simulink model "TEP_Final_NoScript"  (R2024a)
settings: Solver=FixedStepAuto  StartTime=0.0  StopTime=10  FixedStep=1/3600  RelTol=1e-3
model workspace (MAT data in the model file):
  AD : Simulink.Parameter (value not decoded)
  AG : Simulink.Parameter (value not decoded)
  AH : Simulink.Parameter (value not decoded)
  AV : Simulink.Parameter (value not decoded)
  AVP : Simulink.Parameter (value not decoded)
  BCHL : Simulink.Parameter (value not decoded)
  BCHV : Simulink.Parameter (value not decoded)
  BD : Simulink.Parameter (value not decoded)
  BG : Simulink.Parameter (value not decoded)
  BH : Simulink.Parameter (value not decoded)
  BVP : Simulink.Parameter (value not decoded)
  CD : Simulink.Parameter (value not decoded)
  CG : Simulink.Parameter (value not decoded)
  CH : Simulink.Parameter (value not decoded)
  CVP : Simulink.Parameter (value not decoded)
  XMW : Simulink.Parameter (value not decoded)
  XNS : Simulink.Parameter (value not decoded)
  XNSE : Simulink.Parameter (value not decoded)
symbols that are objects in the model workspace (value not decoded): AD, AG, AH, AV, AVP, BD, BG, BH, BVP, CD, CG, CH, CVP, XMW, XNS, XNSE
undefined symbols (not defined in the file or in its folder): magnitude, msgbox, SETPT, XMEAS, XMV
libraries: mylib x360, dspindex x28
(part 7 of 14)

== system TEP_Final_NoScript/Separator/Holdup of Components in Separator/Subsystem3 ==
  Bus Creator : BusCreator  Inputs=8
  Bus Selector3 : BusSelector  OutputSignals=signal1.FCM(I;11)
  FCM(1,11) : Gain
  FCM(2,11) : Gain
  FCM(3,11) : Gain
  FCM(4,11) : Gain
  FCM(5,11) : Gain
  FCM(6,11) : Gain
  FCM(7,11) : Gain
  FCM(8,11) : Gain
  Multiport Selector3 : dspindex/Multiport Selector  rowsOrCols=Rows  idxCellArray={1,2,3,4,5,6,7,8}  idxErrMode=Clip Index
  FCM(I;11) : Outport  VectorParamsAs1DForOutWhenUnconnected=off
  wires:
  Multiport Selector3/3 -> FCM(3,11)/1
  Multiport Selector3/2 -> FCM(2,11)/1
  Multiport Selector3/5 -> FCM(5,11)/1
  Multiport Selector3/8 -> FCM(8,11)/1
  Bus Selector3/1 -> Multiport Selector3/1  "<FCM(I;11)>"
  Multiport Selector3/7 -> FCM(7,11)/1
  Multiport Selector3/6 -> FCM(6,11)/1
  Multiport Selector3/1 -> FCM(1,11)/1
  Multiport Selector3/4 -> FCM(4,11)/1
  [PropertiesStream11] -> Bus Selector3/1
  FCM(5,11)/1 -> Bus Creator/5  "FCM(5;11)"
  FCM(8,11)/1 -> Bus Creator/8  "FCM(8;11)"
  FCM(7,11)/1 -> Bus Creator/7  "FCM(7;11)"
  FCM(6,11)/1 -> Bus Creator/6  "FCM(6;11)"
  FCM(2,11)/1 -> Bus Creator/2  "FCM(2;11)"
  FCM(3,11)/1 -> Bus Creator/3  "FCM(3;11)"
  FCM(4,11)/1 -> Bus Creator/4  "FCM(4;11)"
  FCM(1,11)/1 -> Bus Creator/1  "FCM(1;11)"
  Bus Creator/1 -> FCM(I;11)/1

== system TEP_Final_NoScript/Separator/Holdup of Components in Separator/YP(10) ==
  FCM(1,8) : Inport
  FCM(1,9) : Inport  Port=2
  FCM(1,10) : Inport  Port=3
  FCM(1,11) : Inport  Port=4
  " " : Sum  Inputs=+---
  Bus Selector : BusSelector  OutputSignals=FCM(1;8)
  Bus Selector1 : BusSelector  OutputSignals=FCM(1;9)
  Bus Selector2 : BusSelector  OutputSignals=FCM(1;10)
  Bus Selector3 : BusSelector  OutputSignals=FCM(1;11)
  Integration : mylib/Integration  SystemSampleTime=-1  VariantActivationTime=update diagram  AllowFlexibleInterface=on  Latency=0  AutoFrameSizeCalculation=off
      settings: SourceProductName=TEP Library
  "YY(10) " : Constant  Value=63.75581199
  YY(10) : Outport  VectorParamsAs1DForOutWhenUnconnected=off
  wires:
  "YY(10) "/1 -> Integration/2
  FCM(1,10)/1 -> Bus Selector2/1
  FCM(1,9)/1 -> Bus Selector1/1
  FCM(1,8)/1 -> Bus Selector/1
  " "/1 -> Integration/1
  Integration/1 -> YY(10)/1
  FCM(1,11)/1 -> Bus Selector3/1
  Bus Selector/1 -> " "/1  "<FCM(1;8)>"
  Bus Selector1/1 -> " "/2  "<FCM(1;9)>"
  Bus Selector2/1 -> " "/3  "<FCM(1;10)>"
  Bus Selector3/1 -> " "/4  "<FCM(1;11)>"

== system TEP_Final_NoScript/Separator/Holdup of Components in Separator/YP(11) ==
  FCM(2,8) : Inport
  FCM(2,9) : Inport  Port=2
  FCM(2,10) : Inport  Port=3
  FCM(2,11) : Inport  Port=4
  " " : Sum  Inputs=+---
  Bus Selector : BusSelector  OutputSignals=FCM(2;8)
  Bus Selector1 : BusSelector  OutputSignals=FCM(2;9)
  Bus Selector2 : BusSelector  OutputSignals=FCM(2;10)
  Bus Selector3 : BusSelector  OutputSignals=FCM(2;11)
  Integration : mylib/Integration  SystemSampleTime=-1  VariantActivationTime=update diagram  AllowFlexibleInterface=on  Latency=0  AutoFrameSizeCalculation=off
      settings: SourceProductName=TEP Library
  "YY(11) " : Constant  Value=26.74026066
  YY(11) : Outport  VectorParamsAs1DForOutWhenUnconnected=off
  wires:
  Integration/1 -> YY(11)/1
  FCM(2,8)/1 -> Bus Selector/1
  FCM(2,9)/1 -> Bus Selector1/1
  FCM(2,10)/1 -> Bus Selector2/1
  FCM(2,11)/1 -> Bus Selector3/1
  "YY(11) "/1 -> Integration/2
  " "/1 -> Integration/1
  Bus Selector/1 -> " "/1  "<FCM(2;8)>"
  Bus Selector1/1 -> " "/2  "<FCM(2;9)>"
  Bus Selector2/1 -> " "/3  "<FCM(2;10)>"
  Bus Selector3/1 -> " "/4  "<FCM(2;11)>"

== system TEP_Final_NoScript/Separator/Holdup of Components in Separator/YP(12) ==
  FCM(3,8) : Inport
  FCM(3,9) : Inport  Port=2
  FCM(3,10) : Inport  Port=3
  FCM(3,11) : Inport  Port=4
  " " : Sum  Inputs=+---
  Bus Selector : BusSelector  OutputSignals=FCM(3;11)
  Bus Selector1 : BusSelector  OutputSignals=FCM(3;10)
  Bus Selector2 : BusSelector  OutputSignals=FCM(3;9)
  Bus Selector3 : BusSelector  OutputSignals=FCM(3;8)
  Integration : mylib/Integration  SystemSampleTime=-1  VariantActivationTime=update diagram  AllowFlexibleInterface=on  Latency=0  AutoFrameSizeCalculation=off
      settings: SourceProductName=TEP Library
  "YY(12) " : Constant  Value=46.38532432
  YY(12) : Outport  VectorParamsAs1DForOutWhenUnconnected=off
  wires:
  Integration/1 -> YY(12)/1
  FCM(3,8)/1 -> Bus Selector3/1
  FCM(3,9)/1 -> Bus Selector2/1
  FCM(3,10)/1 -> Bus Selector1/1
  FCM(3,11)/1 -> Bus Selector/1
  " "/1 -> Integration/1
  "YY(12) "/1 -> Integration/2
  Bus Selector3/1 -> " "/1  "<FCM(3;8)>"
  Bus Selector2/1 -> " "/2  "<FCM(3;9)>"
  Bus Selector1/1 -> " "/3  "<FCM(3;10)>"
  Bus Selector/1 -> " "/4  "<FCM(3;11)>"

== system TEP_Final_NoScript/Separator/Holdup of Components in Separator/YP(13) ==
  FCM(4,8) : Inport
  FCM(4,9) : Inport  Port=2
  FCM(4,10) : Inport  Port=3
  FCM(4,11) : Inport  Port=4
  " " : Sum  Inputs=+---
  Bus Selector : BusSelector  OutputSignals=FCM(4;11)
  Bus Selector1 : BusSelector  OutputSignals=FCM(4;10)
  Bus Selector2 : BusSelector  OutputSignals=FCM(4;9)
  Bus Selector3 : BusSelector  OutputSignals=FCM(4;8)
  Integration : mylib/Integration  SystemSampleTime=-1  VariantActivationTime=update diagram  AllowFlexibleInterface=on  Latency=0  AutoFrameSizeCalculation=off
      settings: SourceProductName=TEP Library
  YY(13) : Constant  Value=0.2464521543
  "YY(13) " : Outport  VectorParamsAs1DForOutWhenUnconnected=off
  wires:
  Integration/1 -> "YY(13) "/1
  FCM(4,8)/1 -> Bus Selector3/1
  FCM(4,9)/1 -> Bus Selector2/1
  FCM(4,10)/1 -> Bus Selector1/1
  FCM(4,11)/1 -> Bus Selector/1
  " "/1 -> Integration/1
  YY(13)/1 -> Integration/2
  Bus Selector3/1 -> " "/1  "<FCM(4;8)>"
  Bus Selector2/1 -> " "/2  "<FCM(4;9)>"
  Bus Selector1/1 -> " "/3  "<FCM(4;10)>"
  Bus Selector/1 -> " "/4  "<FCM(4;11)>"

== system TEP_Final_NoScript/Separator/Holdup of Components in Separator/YP(14) ==
  FCM(5,8) : Inport
  FCM(5,9) : Inport  Port=2
  FCM(5,10) : Inport  Port=3
  FCM(5,11) : Inport  Port=4
  " " : Sum  Inputs=+---
  Bus Selector : BusSelector  OutputSignals=FCM(5;8)
  Bus Selector1 : BusSelector  OutputSignals=FCM(5;9)
  Bus Selector2 : BusSelector  OutputSignals=FCM(5;11)
  Bus Selector3 : BusSelector  OutputSignals=FCM(5;10)
  Integration : mylib/Integration  SystemSampleTime=-1  VariantActivationTime=update diagram  AllowFlexibleInterface=on  Latency=0  AutoFrameSizeCalculation=off
      settings: SourceProductName=TEP Library
  YY(14) : Constant  Value=15.20484404
  "YY(14) " : Outport  VectorParamsAs1DForOutWhenUnconnected=off
  wires:
  Integration/1 -> "YY(14) "/1
  FCM(5,8)/1 -> Bus Selector/1
  FCM(5,9)/1 -> Bus Selector1/1
  FCM(5,10)/1 -> Bus Selector3/1
  FCM(5,11)/1 -> Bus Selector2/1
  " "/1 -> Integration/1
  YY(14)/1 -> Integration/2
  Bus Selector/1 -> " "/1  "<FCM(5;8)>"
  Bus Selector1/1 -> " "/2  "<FCM(5;9)>"
  Bus Selector3/1 -> " "/3  "<FCM(5;10)>"
  Bus Selector2/1 -> " "/4  "<FCM(5;11)>"

== system TEP_Final_NoScript/Separator/Holdup of Components in Separator/YP(15) ==
  FCM(6,8) : Inport
  FCM(6,9) : Inport  Port=2
  FCM(6,10) : Inport  Port=3
  FCM(6,11) : Inport  Port=4
  " " : Sum  Inputs=+---
  Bus Selector : BusSelector  OutputSignals=FCM(6;8)
  Bus Selector1 : BusSelector  OutputSignals=FCM(6;11)
  Bus Selector2 : BusSelector  OutputSignals=FCM(6;10)
  Bus Selector3 : BusSelector  OutputSignals=FCM(6;9)
  Integration : mylib/Integration  SystemSampleTime=-1  VariantActivationTime=update diagram  AllowFlexibleInterface=on  Latency=0  AutoFrameSizeCalculation=off
      settings: SourceProductName=TEP Library
  YY(15) : Constant  Value=1.852266172
  "YY(15) " : Outport  VectorParamsAs1DForOutWhenUnconnected=off
  wires:
  Integration/1 -> "YY(15) "/1
  FCM(6,8)/1 -> Bus Selector/1
  FCM(6,9)/1 -> Bus Selector3/1
  FCM(6,10)/1 -> Bus Selector2/1
  FCM(6,11)/1 -> Bus Selector1/1
  " "/1 -> Integration/1
  YY(15)/1 -> Integration/2
  Bus Selector3/1 -> " "/2  "<FCM(6;9)>"
  Bus Selector2/1 -> " "/3  "<FCM(6;10)>"
  Bus Selector1/1 -> " "/4  "<FCM(6;11)>"
  Bus Selector/1 -> " "/1  "<FCM(6;8)>"

== system TEP_Final_NoScript/Separator/Holdup of Components in Separator/YP(16) ==
  FCM(7,8) : Inport
  FCM(7,9) : Inport  Port=2
  FCM(7,10) : Inport  Port=3
  FCM(7,11) : Inport  Port=4
  " " : Sum  Inputs=+---
  Bus Selector : BusSelector  OutputSignals=FCM(7;11)
  Bus Selector1 : BusSelector  OutputSignals=FCM(7;10)
  Bus Selector2 : BusSelector  OutputSignals=FCM(7;9)
  Bus Selector3 : BusSelector  OutputSignals=FCM(7;8)
  Integration : mylib/Integration  SystemSampleTime=-1  VariantActivationTime=update diagram  AllowFlexibleInterface=on  Latency=0  AutoFrameSizeCalculation=off
      settings: SourceProductName=TEP Library
  YY(16) : Constant  Value=52.44639459
  "YY(16) " : Outport  VectorParamsAs1DForOutWhenUnconnected=off
  wires:
  Integration/1 -> "YY(16) "/1
  FCM(7,8)/1 -> Bus Selector3/1
  FCM(7,9)/1 -> Bus Selector2/1
  FCM(7,10)/1 -> Bus Selector1/1
  FCM(7,11)/1 -> Bus Selector/1
  " "/1 -> Integration/1
  YY(16)/1 -> Integration/2
  Bus Selector3/1 -> " "/1  "<FCM(7;8)>"
  Bus Selector2/1 -> " "/2  "<FCM(7;9)>"
  Bus Selector1/1 -> " "/3  "<FCM(7;10)>"
  Bus Selector/1 -> " "/4  "<FCM(7;11)>"

== system TEP_Final_NoScript/Separator/Holdup of Components in Separator/YP(17) ==
  FCM(8,8) : Inport
  FCM(8,9) : Inport  Port=2
  FCM(8,10) : Inport  Port=3
  FCM(8,11) : Inport  Port=4
  " " : Sum  Inputs=+---
  Bus Selector : BusSelector  OutputSignals=FCM(8;11)
  Bus Selector1 : BusSelector  OutputSignals=FCM(8;10)
  Bus Selector2 : BusSelector  OutputSignals=FCM(8;9)
  Bus Selector3 : BusSelector  OutputSignals=FCM(8;8)
  Integration : mylib/Integration  SystemSampleTime=-1  VariantActivationTime=update diagram  AllowFlexibleInterface=on  Latency=0  AutoFrameSizeCalculation=off
      settings: SourceProductName=TEP Library
  YY(17) : Constant  Value=41.20394008
  "YY(17) " : Outport  VectorParamsAs1DForOutWhenUnconnected=off
  wires:
  Integration/1 -> "YY(17) "/1
  FCM(8,8)/1 -> Bus Selector3/1
  FCM(8,9)/1 -> Bus Selector2/1
  FCM(8,10)/1 -> Bus Selector1/1
  " "/1 -> Integration/1
  YY(17)/1 -> Integration/2
  FCM(8,11)/1 -> Bus Selector/1
  Bus Selector3/1 -> " "/1  "<FCM(8;8)>"
  Bus Selector2/1 -> " "/2  "<FCM(8;9)>"
  Bus Selector1/1 -> " "/3  "<FCM(8;10)>"
  Bus Selector/1 -> " "/4  "<FCM(8;11)>"

== system TEP_Final_NoScript/Separator/Pressure of Separator/Subsystem ==
  TCS : Inport
  VVS : Inport  Port=2
  UCVS : Inport  Port=3
  Bus Selector : BusSelector  OutputSignals=UCVS(1),UCVS(2),UCVS(3)
  PPS(1) Partial pressure of Component A mmHg : Product  Inputs=***/
  PPS(2) Partial pressure of Component B mmHg : Product  Inputs=***/
  PPS(3) Partial pressure of Component C mmHg : Product  Inputs=***/
  RG Universal Gas Constant ft³·mmHg/K·lb-mol : Constant  Value=998.9
  TKS Temperature in Separator K : Sum
  To Convert °C to K : Constant  Value=273.15
  PPS(1) : Outport  VectorParamsAs1DForOutWhenUnconnected=off
  PPS(2) : Outport  Port=2  VectorParamsAs1DForOutWhenUnconnected=off
  PPS(3) : Outport  Port=3  VectorParamsAs1DForOutWhenUnconnected=off
  wires:
  Bus Selector/3 -> PPS(3) Partial pressure of Component C mmHg/1  "<UCVS(3)>"
  RG Universal Gas Constant ft³·mmHg/K·lb-mol/1 -> PPS(3) Partial pressure of Component C mmHg/2, PPS(1) Partial pressure of Component A mmHg/2, PPS(2) Partial pressure of Component B mmHg/2
  UCVS/1 -> Bus Selector/1
  Bus Selector/1 -> PPS(1) Partial pressure of Component A mmHg/1  "<UCVS(1)>"
  Bus Selector/2 -> PPS(2) Partial pressure of Component B mmHg/1  "<UCVS(2)>"
  VVS/1 -> PPS(3) Partial pressure of Component C mmHg/4, PPS(2) Partial pressure of Component B mmHg/4, PPS(1) Partial pressure of Component A mmHg/4
  PPS(3) Partial pressure of Component C mmHg/1 -> PPS(3)/1
  To Convert °C to K/1 -> TKS Temperature in Separator K/2
  PPS(1) Partial pressure of Component A mmHg/1 -> PPS(1)/1
  TKS Temperature in Separator K/1 -> PPS(3) Partial pressure of Component C mmHg/3, PPS(2) Partial pressure of Component B mmHg/3, PPS(1) Partial pressure of Component A mmHg/3
  PPS(2) Partial pressure of Component B mmHg/1 -> PPS(2)/1
  TCS/1 -> TKS Temperature in Separator K/1

== system TEP_Final_NoScript/Separator/Pressure of Separator/VPR Vapour Pressure mmHg ==
  TCS : Inport
  AVP(I) Antoine Coefficient A ln(mmHg) : Constant  Value=AVP
  Add : Sum
  Add1 : Sum
  BVP(I) Antoine Coefficient B ln(mmHg)·°C : Constant  Value=BVP
  CVP(I) Antoine Coefficient C °C : Constant  Value=CVP
  Divide : Product  Inputs=*/
  Math Function : Math  SignedPower=on
  VPR : Outport  VectorParamsAs1DForOutWhenUnconnected=off
  wires:
  BVP(I) Antoine Coefficient B ln(mmHg)·°C/1 -> Divide/1
  CVP(I) Antoine Coefficient C °C/1 -> Add/1
  AVP(I) Antoine Coefficient A ln(mmHg)/1 -> Add1/1
  Add/1 -> Divide/2
  Divide/1 -> Add1/2
  Add1/1 -> Math Function/1
  Math Function/1 -> VPR/1
  TCS/1 -> Add/2

== system TEP_Final_NoScript/Separator/Stream 10/HST(10) Molar Enthalpy of Stream 10 MBtu//lb-mol ==
  ITY : Inport
  T : Inport  Port=2
  XST(I,I) : Inport  Port=3
  "Enthalpy of Stream " : mylib/Enthalpy of Stream   SystemSampleTime=-1  VariantActivationTime=update diagram  AllowFlexibleInterface=on  Latency=0  AutoFrameSizeCalculation=off
      settings: SourceProductName=TEP Library
  "H " : Outport  VectorParamsAs1DForOutWhenUnconnected=off
  wires:
  ITY/1 -> "Enthalpy of Stream "/1
  T/1 -> "Enthalpy of Stream "/2
  XST(I,I)/1 -> "Enthalpy of Stream "/3
  "Enthalpy of Stream "/1 -> "H "/1

== system TEP_Final_NoScript/Separator/Stream 10/Subsystem ==
  VPOS(6) : Inport  PortDimensions=1
  Abs : Abs  SaturateOnIntegerOverflow=off
  Constant : Constant  Value=0.0
  Constant1 : Constant  Value=0.151169
  Constant2 : Constant  Value=760
  DLP : Sum  Inputs=+-
  DLP Pressure drop between separator and environment : Merge
  FLMS : Product  Inputs=3
  If : If  IfExpression=u1 < 0
  If Action Subsystem : Subsystem  TreatAsAtomicUnit=on
  If Action Subsystem1 : Subsystem  TreatAsAtomicUnit=on
  Sqrt : Sqrt
  Out1 : Outport  VectorParamsAs1DForOutWhenUnconnected=off
  wires:
  Constant2/1 -> DLP/2
  Constant1/1 -> FLMS/2
  Abs/1 -> Sqrt/1
  DLP Pressure drop between separator and environment/1 -> Abs/1
  [PTS] -> DLP/1
  If Action Subsystem/1(Out1) -> DLP Pressure drop between separator and environment/1
  Constant/1 -> If Action Subsystem/1(In1)
  Sqrt/1 -> FLMS/3
  If Action Subsystem1/1(Out1) -> DLP Pressure drop between separator and environment/2
  If/2 -> If Action Subsystem1/Action
  DLP/1 -> If Action Subsystem1/1(In1), If/1
  VPOS(6)/1 -> FLMS/1
  If/1 -> If Action Subsystem/Action
  FLMS/1 -> Out1/1

== system TEP_Final_NoScript/Separator/Stream 10/XMWS(10) Molecular weight of Stream 10 lb//lb-mol ==
  XST(I,10) : Inport
  Constant : Constant  Value=XMW
  Product : Product
  Sum of Elements : Sum  Inputs=+
  XMWS(10) : Outport  VectorParamsAs1DForOutWhenUnconnected=off
  wires:
  Sum of Elements/1 -> XMWS(10)/1
  Product/1 -> Sum of Elements/1
  XST(I,10)/1 -> Product/1
  Constant/1 -> Product/2

== system TEP_Final_NoScript/Separator/Stream 11/HST(10) Molar Enthalpy of Stream 10 MBtu//lb-mol ==
  ITY : Inport
  T : Inport  Port=2
  XST(I,I) : Inport  Port=3
  "Enthalpy of Stream " : mylib/Enthalpy of Stream   SystemSampleTime=-1  VariantActivationTime=update diagram  AllowFlexibleInterface=on  Latency=0  AutoFrameSizeCalculation=off
      settings: SourceProductName=TEP Library
  "H " : Outport  VectorParamsAs1DForOutWhenUnconnected=off
  wires:
  ITY/1 -> "Enthalpy of Stream "/1
  T/1 -> "Enthalpy of Stream "/2
  XST(I,I)/1 -> "Enthalpy of Stream "/3
  "Enthalpy of Stream "/1 -> "H "/1

== system TEP_Final_NoScript/Separator/Stream 11/PTSL Pressure of Liquid From Separator mmHg ==
  XLS : Inport
  TCS : Inport  Port=2
  Bus Creator1 : BusCreator  Inputs=8
  Demux : Demux  Outputs=8
  PPR(I) : Product
  PTSL Total Pressure of liquid from Separator mmHg : Sum  Inputs=+
  VPR Vapour Pressure mmHg : Subsystem
  PTSL : Outport  PortDimensions=1  VectorParamsAs1DForOutWhenUnconnected=off
  wires:
  Demux/1 -> Bus Creator1/1  "PPR(1)"
  Demux/2 -> Bus Creator1/2  "PPR(2)"
  Demux/7 -> Bus Creator1/7  "PPR(7)"
  TCS/1 -> VPR Vapour Pressure mmHg/1(TCR)
  Demux/8 -> Bus Creator1/8  "PPR(8)"
  PPR(I)/1 -> Demux/1
  VPR Vapour Pressure mmHg/1(VPR) -> PPR(I)/2
  PTSL Total Pressure of liquid from Separator mmHg/1 -> PTSL/1
  XLS/1 -> PPR(I)/1
  Bus Creator1/1 -> PTSL Total Pressure of liquid from Separator mmHg/1
  Demux/6 -> Bus Creator1/6  "PPR(6)"
  Demux/4 -> Bus Creator1/4  "PPR(4)"
  Demux/5 -> Bus Creator1/5  "PPR(5)"
  Demux/3 -> Bus Creator1/3  "PPR(3)"

== system TEP_Final_NoScript/Separator/Stream 9/HST(9) Molar Enthalpy of Stream 9 MBtu//lb-mol ==
  ITY : Inport
  T : Inport  Port=2
  XST(I,I) : Inport  Port=3
  "Enthalpy of Stream " : mylib/Enthalpy of Stream   SystemSampleTime=-1  VariantActivationTime=update diagram  AllowFlexibleInterface=on  Latency=0  AutoFrameSizeCalculation=off
      settings: SourceProductName=TEP Library
  "H " : Outport  PortDimensions=1  VectorParamsAs1DForOutWhenUnconnected=off
  wires:
  ITY/1 -> "Enthalpy of Stream "/1
  T/1 -> "Enthalpy of Stream "/2
  XST(I,I)/1 -> "Enthalpy of Stream "/3
  "Enthalpy of Stream "/1 -> "H "/1

== system TEP_Final_NoScript/Separator/Stream 9/Subsystem ==
  VPOS(5) : Inport
  Abs : Abs  SaturateOnIntegerOverflow=off
  Constant1 : Constant  Value=53.349
  Constant2 : Constant  Value=1E-3
  FLMS : Product  Inputs=3
  "FLMS  " : Merge
  If Action Subsystem2 : Subsystem  TreatAsAtomicUnit=on
  If Action Subsystem3 : Subsystem  TreatAsAtomicUnit=on
  If1 : If  IfExpression=u1 < 1E-3
  Pressure drop : Subsystem
  Sqrt : Sqrt
  Subtract : Sum  Inputs=+-
  "FLMS " : Outport  VectorParamsAs1DForOutWhenUnconnected=off
  wires:
  FLMS/1 -> Subtract/2
  If1/1 -> If Action Subsystem2/Action
  [FLMS] -> Subtract/1
  Subtract/1 -> If Action Subsystem3/1(In1), If1/1
  If Action Subsystem3/1(Out1) -> "FLMS  "/2
  Abs/1 -> Sqrt/1
  Constant1/1 -> FLMS/2
  Sqrt/1 -> FLMS/3
  If1/2 -> If Action Subsystem3/Action
  Constant2/1 -> If Action Subsystem2/1(In1)
  VPOS(5)/1 -> FLMS/1
  If Action Subsystem2/1(Out1) -> "FLMS  "/1
  "FLMS  "/1 -> "FLMS "/1
  Pressure drop/1("DLP ") -> Abs/1

== system TEP_Final_NoScript/Separator/Stream 9/XMWS(9) Molecular weight of Stream 9 lb//lb-mol ==
  XST(I,9) : Inport
  Product : Product
  Sum of Elements : Sum  Inputs=+
  "XMW(I) Molecular weight of components lb/lb-mol " : Constant  Value=[2;25.4;28;32;46;48;62;76]
  XMWS(9) : Outport  VectorParamsAs1DForOutWhenUnconnected=off
  wires:
  Sum of Elements/1 -> XMWS(9)/1
  Product/1 -> Sum of Elements/1
  XST(I,9)/1 -> Product/1
  "XMW(I) Molecular weight of components lb/lb-mol "/1 -> Product/2

== system TEP_Final_NoScript/Separator/Volume of Separator/DLS Molar Density of Liquids in Reactor lb-mol//ft³     ==
  XLS : Inport
  TCS : Inport  Port=2
  "DLS Molar Density of Liquids in Separator lb-mol/ft³ " : Subsystem
  "DLS " : Outport  VectorParamsAs1DForOutWhenUnconnected=off
  wires:
  "DLS Molar Density of Liquids in Separator lb-mol/ft³ "/1("R ") -> "DLS "/1
  TCS/1 -> "DLS Molar Density of Liquids in Separator lb-mol/ft³ "/2(T)
  XLS/1 -> "DLS Molar Density of Liquids in Separator lb-mol/ft³ "/1(X)

== system TEP_Final_NoScript/Stripper/Heat transfer of stripper/If Action Subsystem ==
  In1 : Inport
  Action Port : ActionPort  ActionPortLabel=if(u1 < 100)
  Out1 : Outport  VectorParamsAs1DForOutWhenUnconnected=off
  wires:
  In1/1 -> Out1/1

== system TEP_Final_NoScript/Stripper/Heat transfer of stripper/If Action Subsystem1 ==
  In1 : Inport
  Action Port : ActionPort  ActionPortLabel=else
  Out1 : Outport  VectorParamsAs1DForOutWhenUnconnected=off
  wires:
  In1/1 -> Out1/1

== system TEP_Final_NoScript/Stripper/Holdup of Components in Stripper/Holsup of Liquid Components in Stripper ==
  YY(19:26) : Inport
  Bus Creator : BusCreator  Inputs=8
  Bus Selector : BusSelector  OutputSignals=YY(19),YY(20),YY(21),YY(22),YY(23),YY(24),YY(25),YY(26)
  UCLC(1) Holdup of Component A (Liquid) in Stripper lb-mol : Gain
  UCLC(2) Holdup of Component B (Liquid) in Stripper lb-mol : Gain
  UCLC(3) Holdup of Component C (Liquid) in Stripper lb-mol : Gain
  UCLC(4) Holdup of Component D (Liquid) in Stripper lb-mol : Gain
  UCLC(5) Holdup of Component E (Liquid) in Stripper lb-mol : Gain
  UCLC(6) Holdup of Component F (Liquid) in Stripper lb-mol : Gain
  UCLC(7) Holdup of Component G (Liquid) in Stripper lb-mol : Gain
  UCLC(8) Holdup of Component H (Liquid) in Stripper lb-mol : Gain
  UCLC : Outport  VectorParamsAs1DForOutWhenUnconnected=off
  wires:
  UCLC(8) Holdup of Component H (Liquid) in Stripper lb-mol/1 -> Bus Creator/8
  UCLC(2) Holdup of Component B (Liquid) in Stripper lb-mol/1 -> Bus Creator/2
  UCLC(1) Holdup of Component A (Liquid) in Stripper lb-mol/1 -> Bus Creator/1
  Bus Creator/1 -> UCLC/1
  UCLC(5) Holdup of Component E (Liquid) in Stripper lb-mol/1 -> Bus Creator/5
  UCLC(7) Holdup of Component G (Liquid) in Stripper lb-mol/1 -> Bus Creator/7
  UCLC(4) Holdup of Component D (Liquid) in Stripper lb-mol/1 -> Bus Creator/4
  UCLC(6) Holdup of Component F (Liquid) in Stripper lb-mol/1 -> Bus Creator/6
  UCLC(3) Holdup of Component C (Liquid) in Stripper lb-mol/1 -> Bus Creator/3
  YY(19:26)/1 -> Bus Selector/1
  Bus Selector/1 -> UCLC(1) Holdup of Component A (Liquid) in Stripper lb-mol/1  "<YY(19)>"
  Bus Selector/2 -> UCLC(2) Holdup of Component B (Liquid) in Stripper lb-mol/1  "<YY(20)>"
  Bus Selector/3 -> UCLC(3) Holdup of Component C (Liquid) in Stripper lb-mol/1  "<YY(21)>"
  Bus Selector/4 -> UCLC(4) Holdup of Component D (Liquid) in Stripper lb-mol/1  "<YY(22)>"
  Bus Selector/5 -> UCLC(5) Holdup of Component E (Liquid) in Stripper lb-mol/1  "<YY(23)>"
  Bus Selector/6 -> UCLC(6) Holdup of Component F (Liquid) in Stripper lb-mol/1  "<YY(24)>"
  Bus Selector/7 -> UCLC(7) Holdup of Component G (Liquid) in Stripper lb-mol/1  "<YY(25)>"
  Bus Selector/8 -> UCLC(8) Holdup of Component H (Liquid) in Stripper lb-mol/1  "<YY(26)>"

== system TEP_Final_NoScript/Stripper/Holdup of Components in Stripper/Liquid Component Fraction in Stripper ==
  UTLC : Inport
  UCLC : Inport  Port=2
  Bus Selector : BusSelector  OutputSignals=signal1,signal2,signal3,signal4,signal5,signal6,signal7,signal8
  Mux : Mux  Inputs=8
  XLC(1) : Product  Inputs=*/
  XLC(2) : Product  Inputs=*/
  XLC(3) : Product  Inputs=*/
  XLC(4) : Product  Inputs=*/
  XLC(5) : Product  Inputs=*/
  XLC(6) : Product  Inputs=*/
  XLC(7) : Product  Inputs=*/
  XLC(8) : Product  Inputs=*/
  XLC : Outport  VectorParamsAs1DForOutWhenUnconnected=off
  wires:
  XLC(3)/1 -> Mux/3  "XLC(3)"
  Bus Selector/2 -> XLC(2)/1  "<signal2>"
  Bus Selector/7 -> XLC(7)/1  "<signal7>"
  XLC(5)/1 -> Mux/5  "XLC(5)"
  XLC(7)/1 -> Mux/7  "XLC(7)"
  Bus Selector/3 -> XLC(3)/1  "<signal3>"
  UTLC/1 -> XLC(8)/2, XLC(7)/2, XLC(6)/2, XLC(5)/2, XLC(4)/2, XLC(3)/2, XLC(2)/2, XLC(1)/2
  Bus Selector/6 -> XLC(6)/1  "<signal6>"
  Bus Selector/5 -> XLC(5)/1  "<signal5>"
  XLC(2)/1 -> Mux/2  "XLC(2)"
  XLC(6)/1 -> Mux/6  "XLC(6)"
  Bus Selector/4 -> XLC(4)/1  "<signal4>"
  XLC(1)/1 -> Mux/1  "XLC(1)"
  XLC(8)/1 -> Mux/8  "XLC(8)"
  UCLC/1 -> Bus Selector/1
  XLC(4)/1 -> Mux/4  "XLC(4)"
  Mux/1 -> XLC/1
  Bus Selector/1 -> XLC(1)/1  "<signal1>"
  Bus Selector/8 -> XLC(8)/1  "<signal8>"

== system TEP_Final_NoScript/Stripper/Holdup of Components in Stripper/YP(19) ==
  FCM(1,12) : Inport
  FCM(1,13) : Inport  Port=2
  " " : Sum  Inputs=+-
  Integration : mylib/Integration  SystemSampleTime=-1  VariantActivationTime=update diagram  AllowFlexibleInterface=on  Latency=0  AutoFrameSizeCalculation=off
      settings: SourceProductName=TEP Library
  "YY(19) " : Constant  Value=0.4306056376
  YY(19) : Outport  VectorParamsAs1DForOutWhenUnconnected=off
  wires:
  "YY(19) "/1 -> Integration/2
  FCM(1,13)/1 -> " "/2
  FCM(1,12)/1 -> " "/1
  " "/1 -> Integration/1
  Integration/1 -> YY(19)/1

== system TEP_Final_NoScript/Stripper/Holdup of Components in Stripper/YP(20) ==
  FCM(2,12) : Inport
  FCM(2,13) : Inport  Port=2
  " " : Sum  Inputs=+-
  Integration : mylib/Integration  SystemSampleTime=-1  VariantActivationTime=update diagram  AllowFlexibleInterface=on  Latency=0  AutoFrameSizeCalculation=off
      settings: SourceProductName=TEP Library
  "YY(20) " : Constant  Value=7.9906200783E-3
  YY(20) : Outport  VectorParamsAs1DForOutWhenUnconnected=off
  wires:
  Integration/1 -> YY(20)/1
  FCM(2,12)/1 -> " "/1
  FCM(2,13)/1 -> " "/2
  "YY(20) "/1 -> Integration/2
  " "/1 -> Integration/1

== system TEP_Final_NoScript/Stripper/Holdup of Components in Stripper/YP(21) ==
  FCM(3,12) : Inport
  FCM(3,13) : Inport  Port=2
  " " : Sum  Inputs=+-
  Integration : mylib/Integration  SystemSampleTime=-1  VariantActivationTime=update diagram  AllowFlexibleInterface=on  Latency=0  AutoFrameSizeCalculation=off
      settings: SourceProductName=TEP Library
  "YY(21) " : Constant  Value=0.9056036089
  YY(21) : Outport  VectorParamsAs1DForOutWhenUnconnected=off
  wires:
  Integration/1 -> YY(21)/1
  FCM(3,12)/1 -> " "/1
  FCM(3,13)/1 -> " "/2
  " "/1 -> Integration/1
  "YY(21) "/1 -> Integration/2

== system TEP_Final_NoScript/Stripper/Holdup of Components in Stripper/YP(22) ==
  FCM(4,12) : Inport
  FCM(4,13) : Inport  Port=2
  " " : Sum  Inputs=+-
  Integration : mylib/Integration  SystemSampleTime=-1  VariantActivationTime=update diagram  AllowFlexibleInterface=on  Latency=0  AutoFrameSizeCalculation=off
      settings: SourceProductName=TEP Library
  "YY(22) " : Constant  Value=1.6054258216E-2
  "YY(22)  " : Outport  VectorParamsAs1DForOutWhenUnconnected=off
  wires:
  Integration/1 -> "YY(22)  "/1
  FCM(4,12)/1 -> " "/1
  FCM(4,13)/1 -> " "/2
  " "/1 -> Integration/1
  "YY(22) "/1 -> Integration/2

== system TEP_Final_NoScript/Stripper/Holdup of Components in Stripper/YP(23) ==
  FCM(5,12) : Inport
  FCM(5,13) : Inport  Port=2
  " " : Sum  Inputs=+-
  Integration : mylib/Integration  SystemSampleTime=-1  VariantActivationTime=update diagram  AllowFlexibleInterface=on  Latency=0  AutoFrameSizeCalculation=off
      settings: SourceProductName=TEP Library
  "YY(23) " : Constant  Value=0.7509759687
  "YY(23)  " : Outport  VectorParamsAs1DForOutWhenUnconnected=off
  wires:
  Integration/1 -> "YY(23)  "/1
  FCM(5,12)/1 -> " "/1
  FCM(5,13)/1 -> " "/2
  " "/1 -> Integration/1
  "YY(23) "/1 -> Integration/2

== system TEP_Final_NoScript/Stripper/Holdup of Components in Stripper/YP(24) ==
  FCM(6,12) : Inport
  FCM(6,13) : Inport  Port=2
  " " : Sum  Inputs=+-
  Integration : mylib/Integration  SystemSampleTime=-1  VariantActivationTime=update diagram  AllowFlexibleInterface=on  Latency=0  AutoFrameSizeCalculation=off
      settings: SourceProductName=TEP Library
  YY(24) : Constant  Value=8.8582855955E-2
  "YY(24)  " : Outport  VectorParamsAs1DForOutWhenUnconnected=off
  wires:
  Integration/1 -> "YY(24)  "/1
  FCM(6,12)/1 -> " "/1
  FCM(6,13)/1 -> " "/2
  " "/1 -> Integration/1
  YY(24)/1 -> Integration/2

== system TEP_Final_NoScript/Stripper/Holdup of Components in Stripper/YP(25) ==
  FCM(7,12) : Inport
  FCM(7,13) : Inport  Port=2
  " " : Sum  Inputs=+-
  Integration : mylib/Integration  SystemSampleTime=-1  VariantActivationTime=update diagram  AllowFlexibleInterface=on  Latency=0  AutoFrameSizeCalculation=off
      settings: SourceProductName=TEP Library
  "YY(25) " : Constant  Value=48.27726193
  "YY(25)  " : Outport  VectorParamsAs1DForOutWhenUnconnected=off
  wires:
  Integration/1 -> "YY(25)  "/1
  FCM(7,12)/1 -> " "/1
  FCM(7,13)/1 -> " "/2
  " "/1 -> Integration/1
  "YY(25) "/1 -> Integration/2

== system TEP_Final_NoScript/Stripper/Holdup of Components in Stripper/YP(26) ==
  FCM(8,12) : Inport
  FCM(8,13) : Inport  Port=2
  " " : Sum  Inputs=+-
  Integration : mylib/Integration  SystemSampleTime=-1  VariantActivationTime=update diagram  AllowFlexibleInterface=on  Latency=0  AutoFrameSizeCalculation=off
      settings: SourceProductName=TEP Library
  "YY(26) " : Constant  Value=39.38459028
  "YY(26)   " : Outport  VectorParamsAs1DForOutWhenUnconnected=off
  wires:
  Integration/1 -> "YY(26)   "/1
  FCM(8,12)/1 -> " "/1
  FCM(8,13)/1 -> " "/2
  " "/1 -> Integration/1
  "YY(26) "/1 -> Integration/2

== system TEP_Final_NoScript/Stripper/PTC Pressure of Liquid zone in stripper mmHg/VPR Vapour Pressure mmHg ==
  TCR : Inport
  AVP(I) Antoine Coefficient A ln(mmHg) : Constant  Value=AVP
  Add : Sum
  Add1 : Sum
  BVP(I) Antoine Coefficient B ln(mmHg)·°C : Constant  Value=BVP
  CVP(I) Antoine Coefficient C °C : Constant  Value=CVP
  Divide : Product  Inputs=*/
  Math Function : Math  SignedPower=on
  VPR : Outport  VectorParamsAs1DForOutWhenUnconnected=off
  wires:
  BVP(I) Antoine Coefficient B ln(mmHg)·°C/1 -> Divide/1
  CVP(I) Antoine Coefficient C °C/1 -> Add/1
  AVP(I) Antoine Coefficient A ln(mmHg)/1 -> Add1/1
  Add/1 -> Divide/2
  Divide/1 -> Add1/2
  Add1/1 -> Math Function/1
  Math Function/1 -> VPR/1
  TCR/1 -> Add/2

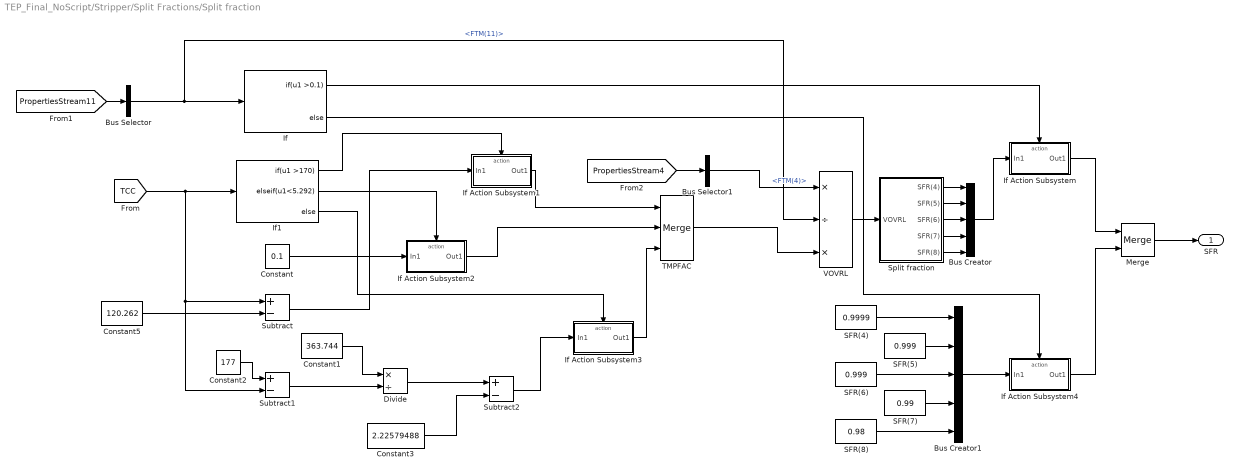
== system TEP_Final_NoScript/Stripper/Split Fractions/Split fraction ==
  Bus Creator : BusCreator  Inputs=5
  Bus Creator1 : BusCreator  Inputs=5
  Bus Selector : BusSelector  OutputSignals=signal1.FTM(11)
  Bus Selector1 : BusSelector  OutputSignals=FTM(4)
  Constant : Constant  Value=0.1
  Constant1 : Constant  Value=363.744
  Constant2 : Constant  Value=177
  Constant3 : Constant  Value=2.22579488
  Constant5 : Constant  Value=120.262
  Divide : Product  Inputs=*/
  If : If  IfExpression=u1 >0.1
  If Action Subsystem : Subsystem  TreatAsAtomicUnit=on
  If Action Subsystem1 : Subsystem  TreatAsAtomicUnit=on
  If Action Subsystem2 : Subsystem  TreatAsAtomicUnit=on
  If Action Subsystem3 : Subsystem  TreatAsAtomicUnit=on
  If Action Subsystem4 : Subsystem  TreatAsAtomicUnit=on
  If1 : If  IfExpression=u1 >170  ElseIfExpressions=u1<5.292
  Merge : Merge
  SFR(4) : Constant  Value=0.9999
  SFR(5) : Constant  Value=0.999
  SFR(6) : Constant  Value=0.999
  SFR(7) : Constant  Value=0.99
  SFR(8) : Constant  Value=0.98
  Split fraction : Subsystem
  Subtract : Sum  Inputs=+-
  Subtract1 : Sum  Inputs=+-
  Subtract2 : Sum  Inputs=+-
  "TMPFAC  " : Merge  Inputs=3
  VOVRL : Product  Inputs=*/*
  SFR : Outport  VectorParamsAs1DForOutWhenUnconnected=off
  wires:
  If/1 -> If Action Subsystem/Action
  Bus Selector/1 -> VOVRL/2, If/1  "<FTM(11)>"
  [TCC] -> If1/1, Subtract1/2, Subtract/1
  Constant5/1 -> Subtract/2
  Constant2/1 -> Subtract1/1
  Subtract1/1 -> Divide/2
  Constant1/1 -> Divide/1
  Divide/1 -> Subtract2/1
  Constant3/1 -> Subtract2/2
  If Action Subsystem1/1(Out1) -> "TMPFAC  "/1
  If Action Subsystem2/1(Out1) -> "TMPFAC  "/2
  If1/1 -> If Action Subsystem1/Action
  Subtract/1 -> If Action Subsystem1/1(In1)
  If1/2 -> If Action Subsystem2/Action
  Constant/1 -> If Action Subsystem2/1(In1)
  Subtract2/1 -> If Action Subsystem3/1(In1)
  If1/3 -> If Action Subsystem3/Action
  If Action Subsystem3/1(Out1) -> "TMPFAC  "/3
  Bus Selector1/1 -> VOVRL/1  "<FTM(4)>"
  "TMPFAC  "/1 -> VOVRL/3
  VOVRL/1 -> Split fraction/1(VOVRL)
  If/2 -> If Action Subsystem4/Action
  Split fraction/1(SFR(4)) -> Bus Creator/1
  Split fraction/2(SFR(5)) -> Bus Creator/2
  Split fraction/3(SFR(6)) -> Bus Creator/3
  Split fraction/4(SFR(7)) -> Bus Creator/4
  Split fraction/5(SFR(8)) -> Bus Creator/5
  Bus Creator/1 -> If Action Subsystem/1(In1)
  Bus Creator1/1 -> If Action Subsystem4/1(In1)
  SFR(4)/1 -> Bus Creator1/1
  SFR(5)/1 -> Bus Creator1/2
  SFR(6)/1 -> Bus Creator1/3
  SFR(7)/1 -> Bus Creator1/4
  SFR(8)/1 -> Bus Creator1/5
  If Action Subsystem4/1(Out1) -> Merge/2
  If Action Subsystem/1(Out1) -> Merge/1
  Merge/1 -> SFR/1
  [PropertiesStream11] -> Bus Selector/1
  [PropertiesStream4] -> Bus Selector1/1

== system TEP_Final_NoScript/Stripper/Stream 12/HST(12) Molar Enthalpy of Stream 12 MBtu//lb-mol ==
  ITY : Inport
  T : Inport  Port=2
  XST(I,I) : Inport  Port=3
  "Enthalpy of Stream " : mylib/Enthalpy of Stream   SystemSampleTime=-1  VariantActivationTime=update diagram  AllowFlexibleInterface=on  Latency=0  AutoFrameSizeCalculation=off
      settings: SourceProductName=TEP Library
  "H " : Outport  VectorParamsAs1DForOutWhenUnconnected=off
  wires:
  ITY/1 -> "Enthalpy of Stream "/1
  T/1 -> "Enthalpy of Stream "/2
  XST(I,I)/1 -> "Enthalpy of Stream "/3
  "Enthalpy of Stream "/1 -> "H "/1

== system TEP_Final_NoScript/Stripper/Stream 13/HST(13) Molar Enthalpy of Stream 13 MBtu//lb-mol ==
  ITY : Inport
  T : Inport  Port=2
  XST(I,I) : Inport  Port=3
  "Enthalpy of Stream " : mylib/Enthalpy of Stream   SystemSampleTime=-1  VariantActivationTime=update diagram  AllowFlexibleInterface=on  Latency=0  AutoFrameSizeCalculation=off
      settings: SourceProductName=TEP Library
  "H " : Outport  VectorParamsAs1DForOutWhenUnconnected=off
  wires:
  ITY/1 -> "Enthalpy of Stream "/1
  T/1 -> "Enthalpy of Stream "/2
  XST(I,I)/1 -> "Enthalpy of Stream "/3
  "Enthalpy of Stream "/1 -> "H "/1

== system TEP_Final_NoScript/Stripper/Stream 5/HST(5) Molar Enthalpy of Stream 5 MBtu//lb-mol ==
  ITY : Inport
  TST(5) : Inport  Port=2
  XST(I,5) : Inport  Port=3
  "Enthalpy of Stream " : mylib/Enthalpy of Stream   SystemSampleTime=-1  VariantActivationTime=update diagram  AllowFlexibleInterface=on  Latency=0  AutoFrameSizeCalculation=off
      settings: SourceProductName=TEP Library
  "H " : Outport  PortDimensions=1  VectorParamsAs1DForOutWhenUnconnected=off
  wires:
  ITY/1 -> "Enthalpy of Stream "/1
  TST(5)/1 -> "Enthalpy of Stream "/2
  XST(I,5)/1 -> "Enthalpy of Stream "/3
  "Enthalpy of Stream "/1 -> "H "/1

== system TEP_Final_NoScript/Stripper/Volume of Stripper/DLC Molar Density of Liquids in Stripper lb-mol//ft³     ==
  XLC : Inport
  TCC : Inport  Port=2
  "DLC Molar Density of Liquids in Stripper lb-mol/ft³ " : Subsystem
  "DLC " : Outport  VectorParamsAs1DForOutWhenUnconnected=off
  wires:
  "DLC Molar Density of Liquids in Stripper lb-mol/ft³ "/1("R ") -> "DLC "/1
  TCC/1 -> "DLC Molar Density of Liquids in Stripper lb-mol/ft³ "/2(T)
  XLC/1 -> "DLC Molar Density of Liquids in Stripper lb-mol/ft³ "/1(X)

== system TEP_Final_NoScript/Subsystem/Braatz/  ==
  XMEAS : Inport
  Bus Selector : BusSelector  OutputSignals=signal1.XMEAS(2),signal8.XMEAS(26)
  CONTROL 1 : Subsystem
  CONTROL 14 : Subsystem
  XMV(1) : Outport  VectorParamsAs1DForOutWhenUnconnected=off
  wires:
  CONTROL 1/1(XMV(1)) -> XMV(1)/1
  CONTROL 14/1(SETPT(1)) -> CONTROL 1/2(SETPT(1))
  XMEAS/1 -> Bus Selector/1
  Bus Selector/1 -> CONTROL 1/1(XMEAS(2))  "<XMEAS(2)>"
  Bus Selector/2 -> CONTROL 14/1(XMEAS(26))  "<XMEAS(26)>"

== system TEP_Final_NoScript/Subsystem/Braatz/ 1 ==
  XMEAS : Inport
  Bus Selector : BusSelector  OutputSignals=signal1.XMEAS(3),signal8.XMEAS(27)
  CONTROL 15 : Subsystem
  CONTROL 2 : Subsystem
  XMV(2) : Outport  VectorParamsAs1DForOutWhenUnconnected=off
  wires:
  CONTROL 2/1(XMV(2)) -> XMV(2)/1
  CONTROL 15/1(SETPT(2)) -> CONTROL 2/2(SETPT(2))
  XMEAS/1 -> Bus Selector/1
  Bus Selector/1 -> CONTROL 2/1(XMEAS(2))  "<XMEAS(3)>"
  Bus Selector/2 -> CONTROL 15/1(XMEAS(27))  "<XMEAS(27)>"

== system TEP_Final_NoScript/Subsystem/Braatz/ 10 ==
  XMEAS : Inport
  Bus Selector : BusSelector  OutputSignals=signal9.XMEAS(30)
  CONTROL 19 : Subsystem
  CONTROL 6 : Subsystem
  XMV(6) : Outport  VectorParamsAs1DForOutWhenUnconnected=off
  wires:
  CONTROL 6/1(XMV(6)) -> XMV(6)/1
  CONTROL 19/1(SETPT(6)) -> CONTROL 6/1(SETPT(6))
  XMEAS/1 -> CONTROL 6/2(XMEAS), Bus Selector/1
  Bus Selector/1 -> CONTROL 19/1(XMEAS(30))  "<XMEAS(30)>"

== system TEP_Final_NoScript/Subsystem/Braatz/ 2 ==
  XMEAS : Inport
  Bus Selector : BusSelector  OutputSignals=signal1.XMEAS(1),signal8.XMEAS(23)
  CONTROL 13 : Subsystem
  CONTROL 3 : Subsystem
  XMV(3) : Outport  VectorParamsAs1DForOutWhenUnconnected=off
  wires:
  CONTROL 3/1(XMV(3)) -> XMV(3)/1
  CONTROL 13/1(SETPT(3)) -> CONTROL 3/2(SETPT(3))
  XMEAS/1 -> Bus Selector/1
  Bus Selector/1 -> CONTROL 3/1(XMEAS(1))  "<XMEAS(1)>"
  Bus Selector/2 -> CONTROL 13/1(XMEAS(23))  "<XMEAS(23)>"

== system TEP_Final_NoScript/Subsystem/Braatz/ 3 ==
  XMEAS : Inport
  Bus Selector : BusSelector  OutputSignals=signal1.XMEAS(4),signal2.XMEAS(8)
  CONTROL 17 : Subsystem
  CONTROL 4 : Subsystem
  XMV(4) : Outport  VectorParamsAs1DForOutWhenUnconnected=off
  wires:
  CONTROL 4/1(XMV(4)) -> XMV(4)/1
  CONTROL 17/1(SETPT(4)) -> CONTROL 4/2(SETPT(4))
  XMEAS/1 -> Bus Selector/1
  Bus Selector/1 -> CONTROL 4/1(XMEAS(4))  "<XMEAS(4)>"
  Bus Selector/2 -> CONTROL 17/1(XMEAS(8))  "<XMEAS(8)>"

== system TEP_Final_NoScript/Subsystem/Braatz/ 4 ==
  XMEAS : Inport
  Bus Selector : BusSelector  OutputSignals=signal1.XMEAS(5)
  CONTROL 5 : Subsystem
  XMV(5) : Outport  VectorParamsAs1DForOutWhenUnconnected=off
  wires:
  CONTROL 5/1(XMV(5)) -> XMV(5)/1
  XMEAS/1 -> Bus Selector/1
  Bus Selector/1 -> CONTROL 5/1(XMEAS(5))  "<XMEAS(5)>"

== system TEP_Final_NoScript/Subsystem/Braatz/ 5 ==
  XMEAS : Inport
  Bus Selector : BusSelector  OutputSignals=signal3.XMEAS(12)
  CONTROL 7 : Subsystem
  XMV(7) : Outport  VectorParamsAs1DForOutWhenUnconnected=off
  wires:
  CONTROL 7/1(XMV(7)) -> XMV(7)/1
  XMEAS/1 -> Bus Selector/1
  Bus Selector/1 -> CONTROL 7/1(XMEAS(12))  "<XMEAS(12)>"

== system TEP_Final_NoScript/Subsystem/Braatz/ 6 ==
  XMEAS : Inport
  Bus Selector : BusSelector  OutputSignals=signal4.XMEAS(15)
  CONTROL 8 : Subsystem
  XMV(8) : Outport  VectorParamsAs1DForOutWhenUnconnected=off
  wires:
  CONTROL 8/1(XMV(8)) -> XMV(8)/1
  XMEAS/1 -> Bus Selector/1
  Bus Selector/1 -> CONTROL 8/1(XMEAS(15))  "<XMEAS(15)>"

== system TEP_Final_NoScript/Subsystem/Braatz/ 7 ==
  XMEAS : Inport
  Bus Selector : BusSelector  OutputSignals=signal4.XMEAS(17)
  CONTROL 11 : Subsystem
  XMV(11) : Outport  VectorParamsAs1DForOutWhenUnconnected=off
  wires:
  CONTROL 11/1(XMV(11)) -> XMV(11)/1
  XMEAS/1 -> Bus Selector/1
  Bus Selector/1 -> CONTROL 11/1(XMEAS(17))  "<XMEAS(17)>"

== system TEP_Final_NoScript/Subsystem/Braatz/ 8 ==
  XMEAS : Inport
  Bus Selector : BusSelector  OutputSignals=XMEAS(21),signal2.XMEAS(9)
  CONTROL 10 : Subsystem
  CONTROL 18 : Subsystem
  XMV(10) : Outport  VectorParamsAs1DForOutWhenUnconnected=off
  wires:
  CONTROL 10/1(XMV(10)) -> XMV(10)/1
  CONTROL 18/1(SETPT(10)) -> CONTROL 10/2(SETPT(10))
  XMEAS/1 -> Bus Selector/1
  Bus Selector/1 -> CONTROL 10/1(XMEAS(21))  "<XMEAS(21)>"
  Bus Selector/2 -> CONTROL 18/1(XMEAS(9))  "<XMEAS(9)>"

== system TEP_Final_NoScript/Subsystem/Braatz/ 9 ==
  XMEAS : Inport
  Bus Selector : BusSelector  OutputSignals=signal4.XMEAS(19),signal4.XMEAS(18),signal10.XMEAS(38)
  CONTROL 16 : Subsystem
  CONTROL 20 : Subsystem
  CONTROL 9 : Subsystem
  XMV(9) : Outport  VectorParamsAs1DForOutWhenUnconnected=off
  wires:
  CONTROL 9/1(XMV(9)) -> XMV(9)/1
  CONTROL 16/1(SETPT(9)) -> CONTROL 9/2(SETPT(9))
  XMEAS/1 -> Bus Selector/1
  Bus Selector/1 -> CONTROL 9/1(XMEAS(19))  "<XMEAS(19)>"
  Bus Selector/2 -> CONTROL 16/1(XMEAS(18))  "<XMEAS(18)>"
  Bus Selector/3 -> CONTROL 20/1(XMEAS(38))  "<XMEAS(38)>"
  CONTROL 20/1(SETPT(16)) -> CONTROL 16/2(SETPT(16))

== system TEP_Final_NoScript/Subsystem1/A and C feed stream/Composition measurement mol% ==
  XST : Inport
  XMNSE : Inport  Port=2
  Bus Creator : BusCreator  Inputs=8
  Subsystem : Subsystem
  SMEASX : Outport
  wires:
  Subsystem/4(SMEASXD) -> Bus Creator/4  "SMEASXD"
  Subsystem/5(SMEASXE) -> Bus Creator/5  "SMEASXE"
  Subsystem/6(SMEASXF) -> Bus Creator/6  "SMEASXF"
  Subsystem/7(SMEASXG) -> Bus Creator/7  "SMEASXG"
  Subsystem/8(SMEASXH) -> Bus Creator/8  "SMEASXH"
  Subsystem/3(SMEASXC) -> Bus Creator/3  "SMEASXC"
  XST/1 -> Subsystem/1(XST)
  Subsystem/2(SMEASXB) -> Bus Creator/2  "SMEASXB"
  Subsystem/1(SMEASXA) -> Bus Creator/1  "SMEASXA"
  Bus Creator/1 -> SMEASX/1  "SMEASX"
  XMNSE/1 -> Subsystem/2(XMNSE)

== system TEP_Final_NoScript/Subsystem1/A and C feed stream/Flow measurement in kg//h ==
  XMEAS in kscmh : Inport
  XST : Inport  Port=2
  " " : Constant  Value=35.3145
  "  " : Constant  Value=0.359
  Convert from lb/h to kg/h : Constant  Value=0.454
  Product : Product  Inputs=3
  XMWS Molecular weight of Stream lb/lb-mol : Subsystem
  lb-mol/h : Product  Inputs=**/
  "SMEASF " : Outport  VectorParamsAs1DForOutWhenUnconnected=off
  wires:
  " "/1 -> lb-mol/h/2
  "  "/1 -> lb-mol/h/3
  XMEAS in kscmh/1 -> lb-mol/h/1
  Convert from lb/h to kg/h/1 -> Product/3
  XST/1 -> XMWS Molecular weight of Stream lb/lb-mol/1(XST)
  lb-mol/h/1 -> Product/2
  XMWS Molecular weight of Stream lb/lb-mol/1(XMWS) -> Product/1
  Product/1 -> "SMEASF "/1  "SMEASF"

== system TEP_Final_NoScript/Subsystem1/A and C feed stream/Pressure measurement in kPa ==
  "P in mm Hg " : Inport
  XMNSE : Inport  Port=2
  " kPa" : Constant  Value=101.325
  " mm Hg   " : Constant  Value=760
  Add : Sum
  Pressure conversion kPa : Product  Inputs=*/*
  SMEASP : Outport  VectorParamsAs1DForOutWhenUnconnected=off
  wires:
  "P in mm Hg "/1 -> Pressure conversion kPa/1
  " kPa"/1 -> Pressure conversion kPa/3
  " mm Hg   "/1 -> Pressure conversion kPa/2
  Pressure conversion kPa/1 -> Add/1
  Add/1 -> SMEASP/1  "SMEASP"
  XMNSE/1 -> Add/2

== system TEP_Final_NoScript/Subsystem1/A and C feed stream/Temperature measurement in C ==
  T in celsius : Inport
  XMNSE : Inport  Port=2
  Add : Sum
  SMEAST : Outport
  wires:
  T in celsius/1 -> Add/1
  Add/1 -> SMEAST/1  "SMEAST"
  XMNSE/1 -> Add/2

== system TEP_Final_NoScript/Subsystem1/A feed stream/Composition measurement mol% ==
  XST : Inport
  XMNSE : Inport  Port=2
  Bus Creator : BusCreator  Inputs=8
  Subsystem : Subsystem
  SMEASX : Outport
  wires:
  Subsystem/4(SMEASXD) -> Bus Creator/4  "SMEASXD"
  Subsystem/5(SMEASXE) -> Bus Creator/5  "SMEASXE"
  Subsystem/6(SMEASXF) -> Bus Creator/6  "SMEASXF"
  Subsystem/7(SMEASXG) -> Bus Creator/7  "SMEASXG"
  Subsystem/8(SMEASXH) -> Bus Creator/8  "SMEASXH"
  Subsystem/3(SMEASXC) -> Bus Creator/3  "SMEASXC"
  XST/1 -> Subsystem/1(XST)
  Subsystem/2(SMEASXB) -> Bus Creator/2  "SMEASXB"
  Subsystem/1(SMEASXA) -> Bus Creator/1  "SMEASXA"
  Bus Creator/1 -> SMEASX/1  "SMEASX"
  XMNSE/1 -> Subsystem/2(XMNSE)

== system TEP_Final_NoScript/Subsystem1/A feed stream/Flow measurement in kg//h ==
  XMEAS in kscmh : Inport
  XST : Inport  Port=2
  " " : Constant  Value=35.3145
  "  " : Constant  Value=0.359
  Convert from lb/h to kg/h : Constant  Value=0.454
  XMWS Molecular weight of Stream lb/lb-mol : Subsystem
  kg/h : Product  Inputs=3
  lb-mol/h : Product  Inputs=**/
  "SMEASF " : Outport  VectorParamsAs1DForOutWhenUnconnected=off
  wires:
  " "/1 -> lb-mol/h/2
  "  "/1 -> lb-mol/h/3
  XMEAS in kscmh/1 -> lb-mol/h/1
  Convert from lb/h to kg/h/1 -> kg/h/3
  XST/1 -> XMWS Molecular weight of Stream lb/lb-mol/1(XST)
  lb-mol/h/1 -> kg/h/2
  XMWS Molecular weight of Stream lb/lb-mol/1(XMWS) -> kg/h/1
  kg/h/1 -> "SMEASF "/1

== system TEP_Final_NoScript/Subsystem1/A feed stream/Pressure measurement in kPa ==
  "P in mm Hg " : Inport
  XMNSE : Inport  Port=2
  " kPa" : Constant  Value=101.325
  " mm Hg   " : Constant  Value=760
  Add : Sum
  Pressure conversion kPa : Product  Inputs=*/*
  SMEASP : Outport  VectorParamsAs1DForOutWhenUnconnected=off
  wires:
  "P in mm Hg "/1 -> Pressure conversion kPa/1
  " kPa"/1 -> Pressure conversion kPa/3
  " mm Hg   "/1 -> Pressure conversion kPa/2
  Pressure conversion kPa/1 -> Add/1
  Add/1 -> SMEASP/1  "SMEASP"
  XMNSE/1 -> Add/2

== system TEP_Final_NoScript/Subsystem1/A feed stream/Temperature measurement in C ==
  T in celsius : Inport
  XMNSE : Inport  Port=2
  Add : Sum
  SMEAST : Outport
  wires:
  T in celsius/1 -> Add/1
  Add/1 -> SMEAST/1  "SMEAST"
  XMNSE/1 -> Add/2

== system TEP_Final_NoScript/Subsystem1/CCIn/Flow measurement in kg//h ==
  XMNSE : Inport
  F in gpm : Inport  Port=2
  Add : Sum
  Product : Product
  Product1 : Product
  gpm to lb/h : Constant  Value=500.72
  kg/kmol : Constant  Value=18.02
  kmol : Constant  Value=0.45359237
  kmol/h : Product
  lb/h to lb-mol/h : Product  Inputs=*/
  lb/lb-mol : Constant  Value=18.02
  "SMEASF " : Outport  VectorParamsAs1DForOutWhenUnconnected=off
  wires:
  Add/1 -> "SMEASF "/1  "SMEASF"
  Product/1 -> Add/1
  XMNSE/1 -> Add/2
  Product1/1 -> lb/h to lb-mol/h/1
  lb/lb-mol/1 -> lb/h to lb-mol/h/2
  lb/h to lb-mol/h/1 -> kmol/h/2
  gpm to lb/h/1 -> Product1/2
  F in gpm/1 -> Product1/1
  kmol/1 -> kmol/h/1
  kmol/h/1 -> Product/1
  kg/kmol/1 -> Product/2

== system TEP_Final_NoScript/Subsystem1/CCIn/Pressure measurement in kPa ==
  XMNSE : Inport
  TC : Inport  Port=2
  A Antoine Coefficient A : Constant  Value=11.6834
  Add : Sum
  Add1 : Sum
  Add2 : Sum  Inputs=+-
  B Antoine Coefficient B : Constant  Value=3816.44
  C Antoine Coefficient C : Constant  Value=-46.13
  Divide : Product  Inputs=*/
  Divide1 : Product  Inputs=**
  Math Function : Math  SignedPower=on
  Temperature in Kelvin K : Sum
  To Convert bar to kPa : Constant  Value=100
  To Convert °C to K : Constant  Value=273.15
  SMEASP : Outport  VectorParamsAs1DForOutWhenUnconnected=off
  wires:
  Add/1 -> SMEASP/1  "SMEASP"
  XMNSE/1 -> Add/2
  To Convert °C to K/1 -> Temperature in Kelvin K/2
  TC/1 -> Temperature in Kelvin K/1
  C Antoine Coefficient C/1 -> Add1/1
  Divide/1 -> Add2/2
  B Antoine Coefficient B/1 -> Divide/1
  Add1/1 -> Divide/2
  Math Function/1 -> Divide1/1
  A Antoine Coefficient A/1 -> Add2/1
  Add2/1 -> Math Function/1
  To Convert bar to kPa/1 -> Divide1/2
  Temperature in Kelvin K/1 -> Add1/2
  Divide1/1 -> Add/1

== system TEP_Final_NoScript/Subsystem1/CCIn/Temperature measurement in C ==
  T in celsius : Inport
  XMNSE : Inport  Port=2
  Add : Sum
  SMEAST : Outport
  wires:
  T in celsius/1 -> Add/1
  Add/1 -> SMEAST/1  "SMEAST"
  XMNSE/1 -> Add/2

== system TEP_Final_NoScript/Subsystem1/CCOut/Pressure measurement in kPa ==
  XMNSE : Inport
  TC : Inport  Port=2
  A Antoine Coefficient A : Constant  Value=11.6834
  Add : Sum
  Add1 : Sum
  Add2 : Sum  Inputs=+-
  B Antoine Coefficient B : Constant  Value=3816.44
  C Antoine Coefficient C : Constant  Value=-46.13
  Divide : Product  Inputs=*/
  Divide1 : Product  Inputs=**
  Math Function : Math  SignedPower=on
  Temperature in Kelvin K : Sum
  To Convert bar to kPa : Constant  Value=100
  To Convert °C to K : Constant  Value=273.15
  SMEASP : Outport  VectorParamsAs1DForOutWhenUnconnected=off
  wires:
  Add/1 -> SMEASP/1  "SMEASP"
  XMNSE/1 -> Add/2
  To Convert °C to K/1 -> Temperature in Kelvin K/2
  TC/1 -> Temperature in Kelvin K/1
  C Antoine Coefficient C/1 -> Add1/1
  Divide/1 -> Add2/2
  B Antoine Coefficient B/1 -> Divide/1
  Add1/1 -> Divide/2
  Math Function/1 -> Divide1/1
  A Antoine Coefficient A/1 -> Add2/1
  Add2/1 -> Math Function/1
  To Convert bar to kPa/1 -> Divide1/2
  Temperature in Kelvin K/1 -> Add1/2
  Divide1/1 -> Add/1

== system TEP_Final_NoScript/Subsystem1/CCOut/Temperature measurement in C ==
  T in celsius : Inport
  XMNSE : Inport  Port=2
  Add : Sum
  SMEAST : Outport
  wires:
  T in celsius/1 -> Add/1
  Add/1 -> SMEAST/1  "SMEAST"
  XMNSE/1 -> Add/2

== system TEP_Final_NoScript/Subsystem1/CCin/Subsystem ==
  Bph : Inport
  FWR in kg/h : Inport  Port=2
  Gain : Gain  Gain=1/3600
  Product : Product
  kg/kmol : Constant  Value=18.02
  kmol to mol : Gain  Gain=1000
  kmol/h : Product  Inputs=*/
  Bphm J/s : Outport  VectorParamsAs1DForOutWhenUnconnected=off
  wires:
  Product/1 -> Gain/1
  kmol/h/1 -> kmol to mol/1
  Bph/1 -> Product/1
  Gain/1 -> Bphm J/s/1
  kg/kmol/1 -> kmol/h/2
  FWR in kg/h/1 -> kmol/h/1
  kmol to mol/1 -> Product/2

== system TEP_Final_NoScript/Subsystem1/CCin/Subsystem1 ==
  T : Inport
  F : Inport  Port=2
  A : Constant  Value=9.069
  Gain : Gain  Gain=1/3600
  J/mol : Product
  Product : Product
  Product1 : Product
  gpm to lb/h : Constant  Value=500.72
  lb/h to lb-mol/h : Product  Inputs=*/
  lb/lb-mol : Constant  Value=18.02
  mol : Constant  Value=453.59
  mol/h : Product
  Q J/s : Outport  VectorParamsAs1DForOutWhenUnconnected=off
  wires:
  A/1 -> J/mol/1
  mol/1 -> mol/h/1
  lb/lb-mol/1 -> lb/h to lb-mol/h/2
  Product1/1 -> lb/h to lb-mol/h/1
  lb/h to lb-mol/h/1 -> mol/h/2
  Product/1 -> Gain/1
  gpm to lb/h/1 -> Product1/2
  Gain/1 -> Q J/s/1
  mol/h/1 -> Product/2
  J/mol/1 -> Product/1
  T/1 -> J/mol/2
  F/1 -> Product1/1
